simulink model "MotorSpeed"  (R2023a)
settings: Solver=VariableStepAuto  StartTime=0.0  StopTime=5.0  RelTol=1e-3
values from neighbouring files (symbols this model uses):
  B = (K*i)/omega    (= 0.00160074422584)    [FreematMotorParameters.m]    (also in MotorVariables02.m = 0.0016)
  J = (-1*(B/s))-(K^2/(s*R))    (= 8.7501592763e-05)    [FreematMotorParameters.m]    (also in MotorVariables02.m = 8.7502e-05)
  K = (1/K_dc)-((i*R)/omega)    (= 0.0620951552979)    [FreematMotorParameters.m]    (also in MotorVariables02.m = 0.0621)
  L = 156.03E-6    (= 0.00015603)    [FreematMotorParameters.m]    (also in MotorVariables02.m = 0.00015604)
  R = 2.93    [FreematMotorParameters.m]    (also in MotorVariables02.m)
settings Model: Creator=NG22  LastModifiedBy=NG22

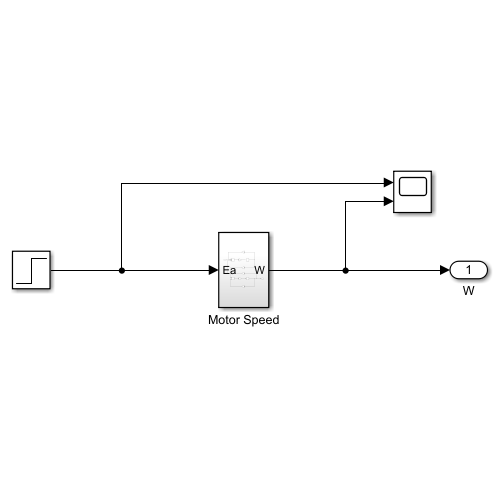
[thumbnail: Simulink's stored preview of the top-level diagram]
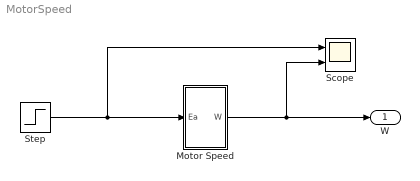
== system MotorSpeed ==
  Motor Speed : Subsystem
  Scope : Scope  NumInputPorts=2
  Step : Step  SampleTime=1
  W : Outport
  wires:
  Step/1 -> Motor Speed/1(Ea), Scope/1
  Motor Speed/1(W) -> Scope/2, W/1

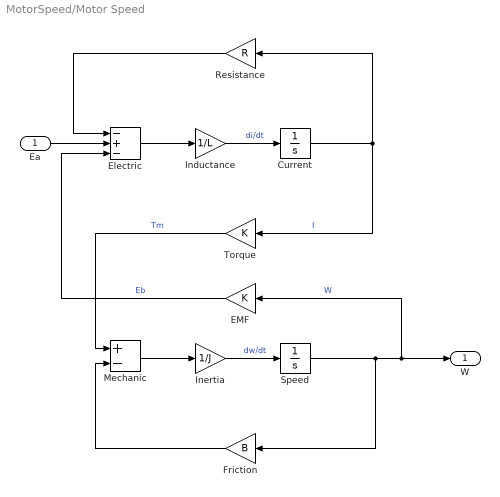
== system MotorSpeed/Motor Speed ==
  Ea : Inport
  "  EMF" : Gain  Gain=K
  Current : Integrator
  Electric : Sum  Inputs=-+-
  Friction : Gain  Gain=B
  Inductance : Gain  Gain=1/L
  Inertia : Gain  Gain=1/J
  Mechanic : Sum  Inputs=+-
  Resistance : Gain  Gain=R
  Speed : Integrator
  Torque : Gain  Gain=K
  W : Outport
  wires:
  Current/1 -> Torque/1, Resistance/1  "I"
  Inductance/1 -> Current/1  "di/dt"
  Speed/1 -> W/1, "  EMF"/1, Friction/1  "W"
  Electric/1 -> Inductance/1
  Inertia/1 -> Speed/1  "dw/dt"
  "  EMF"/1 -> Electric/3  "Eb"
  Resistance/1 -> Electric/1
  Ea/1 -> Electric/2
  Torque/1 -> Mechanic/1  "Tm"
  Friction/1 -> Mechanic/2
  Mechanic/1 -> Inertia/1
